simulink model "IPC4M"  (R2015a)
settings: Solver=ode3  SolverMode=SingleTasking  StartTime=0.0  StopTime=10.0  FixedStep=1e-2  RelTol=1e-7
values from neighbouring files (symbols this model uses):
  d1 = 70    [IPC4Minit.m]
  d2 = 70    [IPC4Minit.m]
  d3 = 70    [IPC4Minit.m]
  d4 = 70    [IPC4Minit.m]
  delta1 = 9    [IPC4Minit.m]
  delta2 = 9    [IPC4Minit.m]
  delta3 = 9    [IPC4Minit.m]
  delta4 = 9    [IPC4Minit.m]
  g = [0;0;-9.81]    [IPC4Minit.m]
  j0 = 10    [IPC4Minit.m]
  j1 = 10    [IPC4Minit.m]
  j1d = 1.00*j1    (= 10)    [IPC4Minit.m]
  j2 = 10    [IPC4Minit.m]
  j2d = 1.00*j2    (= 10)    [IPC4Minit.m]
  j3 = 10    [IPC4Minit.m]
  j3d = 1.00*j3    (= 10)    [IPC4Minit.m]
  j4 = 10    [IPC4Minit.m]
  j4d = 1.00*j4    (= 10)    [IPC4Minit.m]
  k1 = 2000    [IPC4Minit.m]
  k2 = 2000    [IPC4Minit.m]
  k3 = 2000    [IPC4Minit.m]
  k4 = 2000    [IPC4Minit.m]
  kappa1 = 10    [IPC4Minit.m]
  kappa2 = 10    [IPC4Minit.m]
  kappa3 = 10    [IPC4Minit.m]
  kappa4 = 10    [IPC4Minit.m]
  Kc = 150    [IPC4Minit.m]
  l = [1 1 1 1]    [IPC4Minit.m]
  m0 = 10    [IPC4Minit.m]
  m1 = 10    [IPC4Minit.m]
  m1d = 0.00*m1    (= 0)    [IPC4Minit.m]
  m2 = 10    [IPC4Minit.m]
  m2d = 0.00*m2    (= 0)    [IPC4Minit.m]
  m3 = 10    [IPC4Minit.m]
  m3d = 0.00*m3    (= 0)    [IPC4Minit.m]
  m4 = 10    [IPC4Minit.m]
  m4d = 0.00*m4    (= 0)    [IPC4Minit.m]
libraries: aerolibutil x11, dspinverses x3
(part 3 of 3)

== matlab function IPC4M/Interaction dynamics1/MATLAB Function ==
  data: r parameter; A output; x input
function A = ConstraintMatrix(r,x)
A = [-eye(3) skew_sm(quatrot(x(4:7),r(1:3))) eye(3) zeros(3,21);
        zeros(3) -eye(3) zeros(3) eye(3) zeros(3,18);
        -eye(3) skew_sm(quatrot(x(4:7),r(4:6))) zeros(3,6) eye(3) zeros(3,15);
        zeros(3) -eye(3) zeros(3,9) eye(3) zeros(3,12);
        -eye(3) skew_sm(quatrot(x(4:7),r(7:9))) zeros(3,12) eye(3) zeros(3,9);
        zeros(3) -eye(3) zeros(3,15) eye(3) zeros(3,6);
        -eye(3) skew_sm(quatrot(x(4:7),r(10:12))) zeros(3,18) eye(3) zeros(3);
        zeros(3) -eye(3) zeros(3,21) eye(3)];

== matlab function IPC4M/Interaction dynamics1/Centripetal Force ==
  data: dx input; b output; r parameter; x input
function b = centripetalforce(dx,r,x)
b = [skew_sm(dx(4:6))*skew_sm(dx(4:6))*quatrot(x(4:7),r(1:3));
     zeros(3,1);
     skew_sm(dx(4:6))*skew_sm(dx(4:6))*quatrot(x(4:7),r(4:6));
     zeros(3,1);
     skew_sm(dx(4:6))*skew_sm(dx(4:6))*quatrot(x(4:7),r(7:9));
     zeros(3,1);
     skew_sm(dx(4:6))*skew_sm(dx(4:6))*quatrot(x(4:7),r(10:12));
     zeros(3,1)];

== matlab function IPC4M/Interaction dynamics1/Coriolis Force ==
  data: dx input; hcoriolis output; j0 parameter; m0 parameter
function hcoriolis = CoriolisForce(dx,j0,m0)
hcoriolis = [m0*skew_sm(dx(4:6))*dx(1:3);
        j0*skew_sm(dx(4:6))*dx(4:6)];

== matlab function IPC4M/MATLAB Function ==
  data: h_x input; hint output
function hint = InternalForceOpt(h_x)

%External forces: World to object frame
h_xobj = [quatrot(quatconj(x(4:7)')',h_x(1:3));
         h_x(4:6);
         quatrot(quatconj(x(4:7)')',h_x(7:9));
         h_x(10:12);
         quatrot(quatconj(x(4:7)')',h_X(13:15));
         h_x(16:18);
         quatrot(quatconj(x(4:7)')',h_X(19:21));
         h_x(22:24)];
     
%Coordinate Transformation: Object to contact normal frame
%Contact normals
n_obj = r; %Normals in object frame: same direction than virtual stick of contact points
n_con = [0 0 1]';
%Calculation of rotation matrix based on normal in object and contact frame
% Rn = zeros(12,3);
% for i=0:3
%     v = skew_sm(skew_sm(n_con)*n_obj(3*i+1:3*i+3));
%     Rn(3*i+1:3*i+3,1:3) = eye(3) + v + v*v*(1 -n_con*n_obj(3*i+1:3*i+3))/abs(v);
% end
% Quaternion representation of rotation between two vectors: AxisAngle
q = zeros(16);
k = zeros(4);
for i=0:3
    k(i+1) = skew_sm(n_obj(i*3+1:i*3+3))*n_con;
    q(i*4+2:i*4+4) = k(i+1);
    q(i*4+1) = n_obj(i*3+1:i*3+3)'*n_con;
end


% Simplified AxisAngle to Quaternion

%Sum of external and internal forces in object frame
Ared = [-eye(3) skew_sm(r(4:6)-r(1:3)) eye(3) zeros(3,15);
        zeros(3) -eye(3) zeros(3) eye(3) zeros(3,12);
        -eye(3) skew_sm(r(7:9)-r(1:3)) zeros(3,6) eye(3) zeros(3,9);
        zeros(3) -eye(3) zeros(3,9) eye(3) zeros(3,6);
        -eye(3) skew_sm(r(10:12)-r(1:3)) zeros(3,12) eye(3) zeros(3);
        zeros(3) -eye(3) zeros(3,15) eye(3)];

cvx_begin %Call convex optimizer
variable z(18) %Declare z to optimize

%Convert total forces in contact normal frame    
h_obj = h_xobj + Ared'*z;

h_con = zeros(24);
for i=0:3
    h_con(6*i+1:6*i+3) = quatrot(q(4*i+1:4*i+4,h_obj(6*i+1:6*i+3));
    h_con(6*i+4:6*i+6) =  h_obj(6*i+4:6*i+6);
end

S1 = [0 0 1; 0 0 0; 1 0 0; 0 0 0; 0 0 1; 0 1 0; mu*eye(3)];
S2 = [0 0 1; 0 0 0; 1 0 0; 0 0 0; 0 0 1; 0 1 0; mu*eye(3)];
S3 = [0 0 1; 0 0 0; 1 0 0; 0 0 0; 0 0 1; 0 1 0; mu*eye(3)];
S4 = [0 0 1; 0 0 0; 1 0 0; 0 0 0; 0 0 1; 0 1 0; mu*eye(3)];

== matlab function IPC4M/Connecting Spring/ConnectingDamping ==
  data: dx input; h_con output; Dc parameter
function h_con = ConnectingDamping(dx,Dc)

H = kron([0.75 -0.25 -0.25 -0.25; -0.25 0.75 -0.25 -0.25; -0.25 -0.25 0.75 -0.25; -0.25 -0.25 -0.25 0.75],eye(3));
v_o = [eye(3) zeros(3) eye(3) zeros(3) eye(3) zeros(3) eye(3) zeros(3)] * dx;
v = [dx(1:3);dx(7:9);dx(13:15);dx(19:21)];
deltav = v - [eye(3);eye(3);eye(3);eye(3)]*v_o;
dmp = Dc*[deltav(1:3);
          deltav(4:6);
          deltav(7:9);
          deltav(10:12)];
f_con = H*dmp;
h_con = [f_con(1:3);zeros(3,1);f_con(4:6);zeros(3,1);f_con(7:9);zeros(3,1);f_con(10:12);zeros(3,1)];

== matlab function IPC4M/Connecting Spring/ConnectingStiffness ==
  data: x input; h_con output; l parameter; Kc parameter
function h_con = ConnectingStiffness(x,l,Kc)

H = kron([0.75 -0.25 -0.25 -0.25; -0.25 0.75 -0.25 -0.25; -0.25 -0.25 0.75 -0.25; -0.25 -0.25 -0.25 0.75],eye(3));
p_o = [eye(3) zeros(3,4) eye(3) zeros(3,4) eye(3) zeros(3,4) eye(3) zeros(3,4)] * x;
p = [x(1:3);x(8:10);x(15:17);x(22:24)];
deltap = p - [eye(3);eye(3);eye(3);eye(3)]*p_o;
stf = Kc*[(norm(deltap(1:3))-l(1))/norm(deltap(1:3))*deltap(1:3);
          (norm(deltap(4:6))-l(2))/norm(deltap(4:6))*deltap(4:6);
          (norm(deltap(7:9))-l(3))/norm(deltap(7:9))*deltap(7:9);
          (norm(deltap(10:12))-l(4))/norm(deltap(10:12))*deltap(10:12)];
f_con = H*stf;
h_con = [f_con(1:3);zeros(3,1);f_con(4:6);zeros(3,1);f_con(7:9);zeros(3,1);f_con(10:12);zeros(3,1)];

== matlab function IPC4M/Kinematic Coordination/Grasp Matrix ==
  data: r parameter; G output; x input
function G = GraspMatrix(r,x)
x_o = [eye(3) zeros(3,4) eye(3) zeros(3,4) eye(3) zeros(3,4) eye(3) zeros(3,4)] * x;
G = [eye(3) zeros(3) eye(3) zeros(3) eye(3) zeros(3) eye(3) zeros(3);
    skew_sm(quatrot(x(4:7),x(1:3)-x_o)) eye(3) skew_sm(quatrot(x(4:7),x(8:10)-x_o)) eye(3) skew_sm(quatrot(x(4:7),x(15:17)-x_o)) eye(3) skew_sm(quatrot(x(4:7),x(22:24)-x_o)) eye(3)];

== matlab function IPC4M/Kinematic Coordination/Manipulator Position//Orientation in World Frame ==
  data: p_do input; q_do input; x_d output; r parameter
function x_d = manipulatorpose(p_do,q_do,r)

x_d = [p_do + quatrot(q_do,r(1:3));
        q_do;
        p_do + quatrot(q_do,r(4:6));
        q_do;
        p_do + quatrot(q_do,r(7:9));
        q_do;
        p_do + quatrot(q_do,r(10:12));
        q_do];

== matlab function IPC4M/Kinematic Coordination/Centripetal Force ==
  data: dx_do input; b output; x input
function b = centripetalforce(dx_do,x)
x_o = [eye(3) zeros(3,4) eye(3) zeros(3,4) eye(3) zeros(3,4) eye(3) zeros(3,4)] * x;
b = [skew_sm(dx_do(4:6))*skew_sm(dx_do(4:6))*quatrot(x(4:7),x(1:3)-x_o);
     zeros(3,1);
     skew_sm(dx_do(4:6))*skew_sm(dx_do(4:6))*quatrot(x(4:7),x(8:10)-x_o);
     zeros(3,1);
     skew_sm(dx_do(4:6))*skew_sm(dx_do(4:6))*quatrot(x(4:7),x(15:17)-x_o);
     zeros(3,1);
     skew_sm(dx_do(4:6))*skew_sm(dx_do(4:6))*quatrot(x(4:7),x(22:24)-x_o);
     zeros(3,1)];

== matlab function IPC4M/Inverse Dynamics/MATLAB Function3 ==
  data: r parameter; G output; x input
function G = GraspMatrix(r,x)
G = [eye(3) zeros(3) eye(3) zeros(3) eye(3) zeros(3) eye(3) zeros(3);
    skew_sm(quatrot(x(4:7),r(1:3))) eye(3) skew_sm(quatrot(x(4:7),r(4:6))) eye(3) skew_sm(quatrot(x(4:7),r(7:9))) eye(3) skew_sm(quatrot(x(4:7),r(10:12))) eye(3)];

== matlab function IPC4M/Impedance control/Manipulator1/k1; 2kappa1*eta1 ==
  data: eta1 input; K output; k1 parameter; kappa1 parameter
function K = stiffness(eta1,k1,kappa1)
K = blkdiag(k1*eye(3),2*eta1*kappa1*eye(3));

== matlab function IPC4M/Impedance control/Manipulator2/MATLAB Function1 ==
  data: eta2 input; K output; k2 parameter; kappa2 parameter
function K = stiffness(eta2,k2,kappa2)
K = blkdiag(k2*eye(3),2*eta2*kappa2*eye(3));

== matlab function IPC4M/Impedance control/Manipulator3/MATLAB Function2 ==
  data: eta3 input; K output; k3 parameter; kappa3 parameter
function K = stiffness(eta3,k3,kappa3)
K = blkdiag(k3*eye(3),2*eta3*kappa3*eye(3));

== matlab function IPC4M/Impedance control/Manipulator4/MATLAB Function3 ==
  data: eta4 input; K output; k4 parameter; kappa4 parameter
function K = stiffness(eta4,k4,kappa4)
K = blkdiag(k4*eye(3),2*eta4*kappa4*eye(3));

== matlab function IPC4M/Manipulator dynamics/Reduced Constraint Matrix ==
  data: r parameter; Ared output; x input
function Ared = ReducedConstraintMAtrix(r,x)
%x_o = [eye(3) zeros(3,4) eye(3) zeros(3,4) eye(3) zeros(3,4) eye(3) zeros(3,4)] * x;
Ared = [-eye(3) skew_sm(quatrot(x(4:7),r(4:6)-r(1:3))) eye(3) zeros(3,15);
        zeros(3) -eye(3) zeros(3) eye(3) zeros(3,12);
        -eye(3) skew_sm(quatrot(x(4:7),r(7:9)-r(1:3))) zeros(3,6) eye(3) zeros(3,9);
        zeros(3) -eye(3) zeros(3,9) eye(3) zeros(3,6);
        -eye(3) skew_sm(quatrot(x(4:7),r(10:12)-r(1:3))) zeros(3,12) eye(3) zeros(3);
        zeros(3) -eye(3) zeros(3,15) eye(3)];
% Ared = [-eye(3) skew_sm(quatrot(x(4:7),x(8:10)-x(1:3))) eye(3) zeros(3,15);
%         zeros(3) -eye(3) zeros(3) eye(3) zeros(3,12);
%         -eye(3) skew_sm(quatrot(x(4:7),x(15:17)-x(1:3))) zeros(3,6) eye(3) zeros(3,9);
%         zeros(3) -eye(3) zeros(3,9) eye(3) zeros(3,6);
%         -eye(3) skew_sm(quatrot(x(4:7),x(22:24)-x(1:3))) zeros(3,12) eye(3) zeros(3);
%         zeros(3) -eye(3) zeros(3,15) eye(3)];

== matlab function IPC4M/Manipulator dynamics/Centripal Force ==
  data: r parameter; x input; bred output; dx input
function bred = ReducedCentripetalvector(r,x,dx)
bred = [skew_sm(dx(4:6))*skew_sm(dx(4:6))*quatrot(x(4:7),(r(4:6)-r(1:3)));
        zeros(3,1);
        skew_sm(dx(4:6))*skew_sm(dx(4:6))*quatrot(x(4:7),(r(7:9)-r(1:3)));
        zeros(3,1);
        skew_sm(dx(4:6))*skew_sm(dx(4:6))*quatrot(x(4:7),(r(10:12)-r(1:3)));
        zeros(3,1)];
%     bred = [skew_sm(dx(4:6))*skew_sm(dx(4:6))*quatrot(x(4:7),(x(8:10)-x(1:3)));
%         zeros(3,1);
%         skew_sm(dx(4:6))*skew_sm(dx(4:6))*quatrot(x(4:7),(x(15:17)-x(1:3)));
%         zeros(3,1);
%         skew_sm(dx(4:6))*skew_sm(dx(4:6))*quatrot(x(4:7),(x(22:24)-x(1:3)));
%         zeros(3,1)];

== matlab function IPC4M/Interaction dynamics/Apparent Inertia ==
  data: G input; Mapp output; M input; m0 parameter; j0 parameter
function Mapp = ApparentInertia(G,M,m0,j0)
Mapp = blkdiag(m0*eye(3),j0*eye(3)) + G*M*G';

== matlab function IPC4M/Interaction dynamics/Grasp Matrix ==
  data: r parameter; G output; x input
function G = GraspMatrix(r,x)
G = [eye(3) zeros(3) eye(3) zeros(3) eye(3) zeros(3) eye(3) zeros(3);
    skew_sm(quatrot(x(4:7),r(1:3))) eye(3) skew_sm(quatrot(x(4:7),r(4:6))) eye(3) skew_sm(quatrot(x(4:7),r(7:9))) eye(3) skew_sm(quatrot(x(4:7),r(10:12))) eye(3)];

== matlab function IPC4M/Interaction dynamics/Coriolis Force ==
  data: dx input; hcoriolis output; j0 parameter; m0 parameter
function hcoriolis = CoriolisForce(dx,j0,m0)
hcoriolis = [m0*skew_sm(dx(4:6))*dx(1:3);
        j0*skew_sm(dx(4:6))*dx(4:6)];

== matlab function IPC4M/Interaction dynamics/Centripetal Force ==
  data: dx input; b output; r parameter; x input
function b = centripetalforce(dx,r,x)
b = [skew_sm(dx(4:6))*skew_sm(dx(4:6))*quatrot(x(4:7),r(1:3));
     zeros(3,1);
     skew_sm(dx(4:6))*skew_sm(dx(4:6))*quatrot(x(4:7),r(4:6));
     zeros(3,1);
     skew_sm(dx(4:6))*skew_sm(dx(4:6))*quatrot(x(4:7),r(7:9));
     zeros(3,1);
     skew_sm(dx(4:6))*skew_sm(dx(4:6))*quatrot(x(4:7),r(10:12));
     zeros(3,1)];

== matlab function IPC4M/Manipulator motion/Grasp Matrix ==
  data: r parameter; G output; x input
function G = GraspMatrix(r,x)
G = [eye(3) zeros(3) eye(3) zeros(3) eye(3) zeros(3) eye(3) zeros(3);
    skew_sm(quatrot(x(4:7),r(1:3))) eye(3) skew_sm(quatrot(x(4:7),r(4:6))) eye(3) skew_sm(quatrot(x(4:7),r(7:9))) eye(3) skew_sm(quatrot(x(4:7),r(10:12))) eye(3)];

== matlab function IPC4M/Manipulator motion/Manipualtor pose in world frame ==
  data: p_o input; q_o input size=4; x output; r parameter
function x = manipulatorpose(p_o,q_o,r)

x = [p_o + quatrot(q_o,r(1:3));
        q_o;
        p_o + quatrot(q_o,r(4:6));
        q_o;
        p_o + quatrot(q_o,r(7:9));
        q_o;
        p_o + quatrot(q_o,r(10:12));
        q_o ];

== matlab function IPC4M/Nullspace/Reduced Constraint Matrix ==
  data: r parameter; Ared output; x input
function Ared = ReducedConstraintMAtrix(r,x)
Ared = [-eye(3) skew_sm(quatrot(x(4:7),r(4:6)-r(1:3))) eye(3) zeros(3,15);
        zeros(3) -eye(3) zeros(3) eye(3) zeros(3,12);
        -eye(3) skew_sm(quatrot(x(4:7),r(7:9)-r(1:3))) zeros(3,6) eye(3) zeros(3,9);
        zeros(3) -eye(3) zeros(3,9) eye(3) zeros(3,6);
        -eye(3) skew_sm(quatrot(x(4:7),r(10:12)-r(1:3))) zeros(3,12) eye(3) zeros(3);
        zeros(3) -eye(3) zeros(3,15) eye(3)];

== matlab function IPC4M/Allocator/MATLAB Function1 ==
  data: r parameter; bred output; dx input; x input
function bred = ReducedCentripetalvector(r,dx,x)
% bred = [skew_sm(dx(4:6))*skew_sm(dx(4:6))*quatrot(x(4:7),r(4:6)-r(1:3));
%     zeros(3,1);
%     skew_sm(dx(4:6))*skew_sm(dx(4:6))*quatrot(x(4:7),r(7:9)-r(1:3));
%     zeros(3,1);
%     skew_sm(dx(4:6))*skew_sm(dx(4:6))*quatrot(x(4:7),r(10:12)-r(1:3));
%     zeros(3,1)];
    bred = [skew_sm(dx(4:6))*skew_sm(dx(4:6))*quatrot(x(4:7),(x(8:10)-x(1:3)));
        zeros(3,1);
        skew_sm(dx(4:6))*skew_sm(dx(4:6))*quatrot(x(4:7),(x(15:17)-x(1:3)));
        zeros(3,1);
        skew_sm(dx(4:6))*skew_sm(dx(4:6))*quatrot(x(4:7),(x(22:24)-x(1:3)));
        zeros(3,1)];

== matlab function IPC4M/Allocator/MATLAB Function ==
  data: r parameter; Ared output; x input
function Ared = ReducedConstraintMAtrix(r,x)
% Ared = [-eye(3) skew_sm(quatrot(x(4:7),r(4:6)-r(1:3))) eye(3) zeros(3,15);
%         zeros(3) -eye(3) zeros(3) eye(3) zeros(3,12);
%         -eye(3) skew_sm(quatrot(x(4:7),r(7:9)-r(1:3))) zeros(3,6) eye(3) zeros(3,9);
%         zeros(3) -eye(3) zeros(3,9) eye(3) zeros(3,6);
%         -eye(3) skew_sm(quatrot(x(4:7),r(10:12)-r(1:3))) zeros(3,12) eye(3) zeros(3);
%         zeros(3) -eye(3) zeros(3,15) eye(3)];
Ared = [-eye(3) skew_sm(quatrot(x(4:7),x(8:10)-x(1:3))) eye(3) zeros(3,15);
        zeros(3) -eye(3) zeros(3) eye(3) zeros(3,12);
        -eye(3) skew_sm(quatrot(x(4:7),x(15:17)-x(1:3))) zeros(3,6) eye(3) zeros(3,9);
        zeros(3) -eye(3) zeros(3,9) eye(3) zeros(3,6);
        -eye(3) skew_sm(quatrot(x(4:7),x(22:24)-x(1:3))) zeros(3,12) eye(3) zeros(3);
        zeros(3) -eye(3) zeros(3,15) eye(3)];

== matlab function IPC4M/Object to World Frame ==
  data: z input; x input; z_w output
function z_w = object2worldFrame(z,x)

z_w = [quatrot(x(4:7),z(1:3));
       z(4:6);
       quatrot(x(4:7),z(7:9));
       z(10:12);
       quatrot(x(4:7),z(13:15));
       z(16:18)];

== matlab function IPC4M/Manipulator dynamics/World to Object Frame ==
  data: hw input; x input; h_int output
function h_int = inertial2objectFrame(hw,x)

h_int = [quatrot(quatconj(x(4:7)')',hw(1:3));
         hw(4:6);%quatrot(quatconj(x(4:7)')',hw(4:6));
         quatrot(quatconj(x(4:7)')',hw(7:9));
         hw(10:12);%quatrot(quatconj(x(4:7)')',hw(10:12));
         quatrot(quatconj(x(4:7)')',hw(13:15));
         hw(16:18);%quatrot(quatconj(x(4:7)')',hw(16:18));
         quatrot(quatconj(x(4:7)')',hw(19:21));
         hw(22:24)];%quatrot(quatconj(x(4:7)')',hw(22:24));];
